simulink model "Esercitazione5_sim"  (R2020b)
settings: Solver=VariableStepAuto  StartTime=0.0  StopTime=15  RelTol=1e-3
values from neighbouring files (symbols this model uses):
  sys_d = c2d(sys_c,Tcampion, 'zoh')    [Esercizio5.m]    (also in myESE4.m = c2d(sys_G,Tc, 'zoh'))
  Tcampion = 1/10    (= 0.1)    [Esercizio5.m]
settings Model: Creator=chiar  LastModifiedBy=chiar

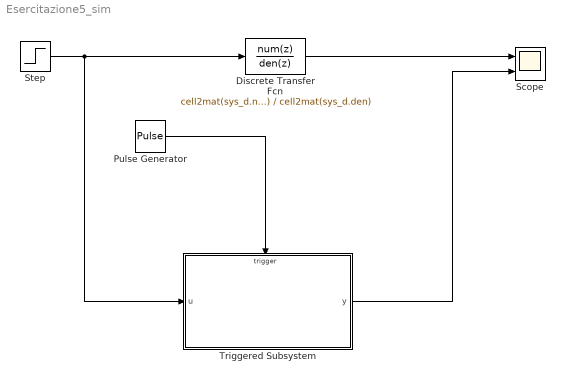
== system Esercitazione5_sim ==
  Discrete Transfer Fcn : DiscreteTransferFcn  Numerator=cell2mat(sys_d.num)  Denominator=cell2mat(sys_d.den)  SampleTime=Tcampion
  Pulse Generator : DiscretePulseGenerator  PulseType=Time based  Period=Tcampion  PulseWidth=5
  Scope : Scope  NumInputPorts=2
  Step : Step  SampleTime=0
  Triggered Subsystem : Subsystem  TreatAsAtomicUnit=on
  wires:
  Step/1 -> Triggered Subsystem/1(u), Discrete Transfer Fcn/1
  Discrete Transfer Fcn/1 -> Scope/1
  Pulse Generator/1 -> Triggered Subsystem/Trigger
  Triggered Subsystem/1(y) -> Scope/2

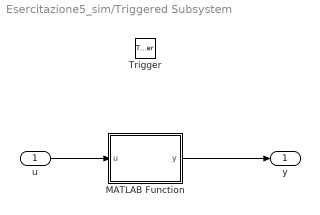
== system Esercitazione5_sim/Triggered Subsystem ==
  u : Inport
  Trigger : TriggerPort  VariantControl=Variant
  MATLAB Function : MATLAB Function  TreatAsAtomicUnit=on
  y : Outport
  wires:
  u/1 -> MATLAB Function/1(u)
  MATLAB Function/1(y) -> y/1

== matlab function Esercitazione5_sim/Triggered Subsystem/MATLAB Function ==
  data: u input; y output
function y = fcn(u)

%Scrivo l'equazione alle differenze che ho ricavato su quaderno

%Definisco le variabili PERSISTENT per renderle dotate di memoria e poter
%usare il valore per passi successivi

persistent ym1 ym2 um1 um2

%% 
%Definisco cosa succede all'istente 0

if isempty(ym1) %Se è vuota una delle variabili, inizializzo tutto a 0
    ym1=0;
    ym2=0;
    um1=0;
    um2=0;
end

%%
%Ricavo i coefficienti digitando cell2mat(sys.den)e sys.num per
%visualiazzare i coefficienti

%Per avere tanti decimali, digito formato long

%NB: metto solo i moduli dei coefficienti!

d1= 1.856066842536674 ;
d0= 0.860707976425058;
n1= 0.466298633682076 ;
n0= 0.461657499793692;


y = d1*ym1-d0*ym2+n1*um1-n0*um2;

%%
%Preparo la funzione per l'istante successivo

ym2=ym1;
ym1=y;

um2=um1;
um1=u;
